simulink model "wi_dac_cad"  (R2023b)
settings: Solver=VariableStepAuto  StartTime=0.0  StopTime=10.0  RelTol=1e-3
values from neighbouring files (symbols this model uses):
  final_value = 150    [test.m]
  Hp = Kp /( Tp *s  +1)    [test.m]
  Hpi = Hee * Hp2    [test.m]
  Hr = Hd/ Hf    [test.m]
  Hri = ( 97.67 * s + 1 ) / (12.33*s)    [test.m]
  initial_value = 25    [test.m]
  step_time = 10    [test.m]
undefined symbols (not defined in the file or in its folder): rez
libraries: fl_lib x10
settings Model: Creator=wombelbat  LastModifiedBy=wombelbat

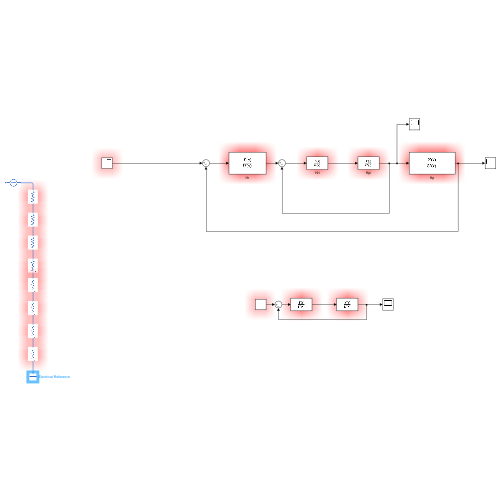
[thumbnail: Simulink's stored preview of the top-level diagram]
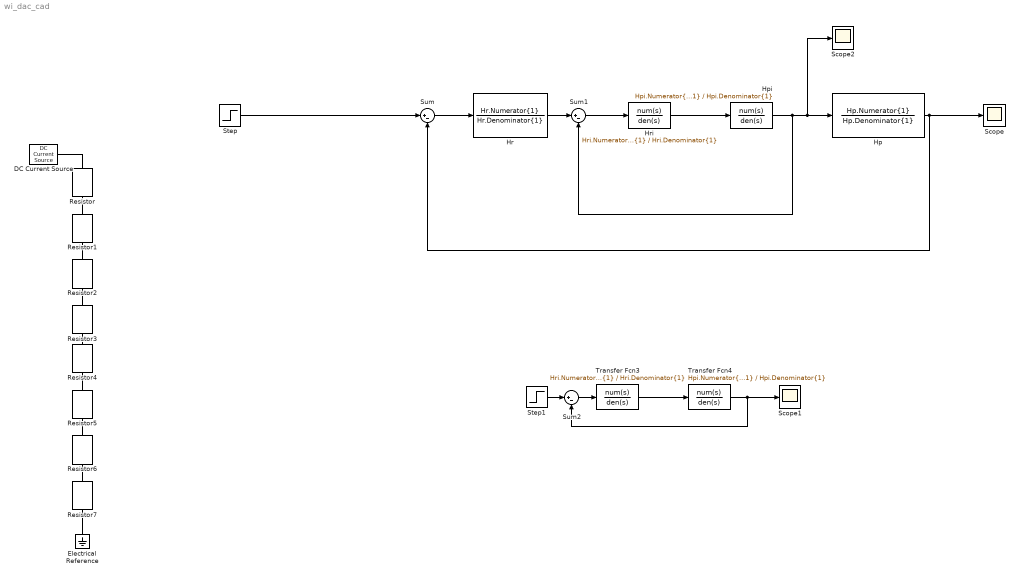
== system wi_dac_cad ==
  DC Current Source : fl_lib/Electrical/Electrical Sources/DC Current Source  i0=1 A
      settings: InternalSimscapePortConfiguration="{\"Bottom\":[],\"Left\":[{\"id\":\"p\",\"label\":\"\",\"type\":\"foundation.electrical.electrical\"}],\"Right\":[{\"id\":\"n\",\"label\":\"\",\"type\":\"foundation.electrical.electrical\"}],\"Top\":[]}"
  Electrical Reference : fl_lib/Electrical/Electrical Elements/Electrical Reference
  Hp : TransferFcn  Numerator=Hp.Numerator{1}  Denominator=Hp.Denominator{1}
  Hpi : TransferFcn  Numerator=Hpi.Numerator{1}  Denominator=Hpi.Denominator{1}
  Hr : TransferFcn  Numerator=Hr.Numerator{1}  Denominator=Hr.Denominator{1}
  Hri : TransferFcn  Numerator=Hri.Numerator{1}  Denominator=Hri.Denominator{1}
  Resistor{,1..7} (8 alike) : fl_lib/Electrical/Electrical Elements/Resistor  R=rez Ohm  i_specify=off  i_priority=None  i=0 A  i_nominal_specify=off  i_nominal_unit=A  i_nominal_value=1  v_specify=off  v_priority=None  v=0 V  v_nominal_specify=off  v_nominal_unit=V  v_nominal_value=1
  Scope : Scope
  Scope1 : Scope
  Scope2 : Scope
  Step : Step  Time=step_time  Before=initial_value  After=final_value  SampleTime=0
  Step1 : Step  Time=step_time  Before=initial_value  After=final_value  SampleTime=0
  Sum : Sum  Inputs=|+-
  Sum1 : Sum  Inputs=|+-
  Sum2 : Sum  Inputs=|+-
  Transfer Fcn3 : TransferFcn  Numerator=Hri.Numerator{1}  Denominator=Hri.Denominator{1}
  Transfer Fcn4 : TransferFcn  Numerator=Hpi.Numerator{1}  Denominator=Hpi.Denominator{1}
  wires:
  Step1/1 -> Sum2/1
  Transfer Fcn4/1 -> Scope1/1, Sum2/2
  Sum1/1 -> Hri/1
  Hp/1 -> Sum/2, Scope/1
  Step/1 -> Sum/1
  Sum/1 -> Hr/1
  Sum2/1 -> Transfer Fcn3/1
  Transfer Fcn3/1 -> Transfer Fcn4/1
  Hri/1 -> Hpi/1
  Hpi/1 -> Scope2/1, Hp/1, Sum1/2
  Hr/1 -> Sum1/1
  connections:
  Resistor2/LConn1 -- Resistor1/RConn1
  Resistor6/LConn1 -- Resistor5/RConn1
  Resistor4/LConn1 -- Resistor3/RConn1
  Resistor/RConn1 -- Resistor1/LConn1
  Resistor2/RConn1 -- Resistor3/LConn1
  Resistor4/RConn1 -- Resistor5/LConn1
  Resistor6/RConn1 -- Resistor7/LConn1
  DC Current Source/LConn1 -- Resistor/LConn1
  Electrical Reference/LConn1 -- Resistor7/RConn1
